simulink model "chap6_8sim"  (Simulink 5.0)
settings: Solver=ode45  StartTime=0.0  StopTime=20  RelTol=1e-3
libraries: simulink x1
settings Model: LastModifiedBy=Administrator

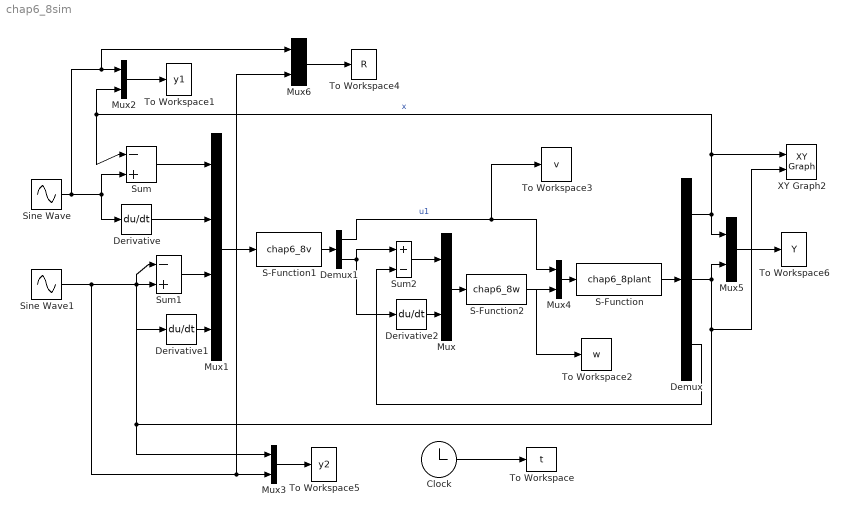
== system chap6_8sim ==
  Clock : Clock
  Demux : Demux  Outputs=3
  Demux1 : Demux  Outputs=2
  Derivative : Derivative
  Derivative1 : Derivative
  Derivative2 : Derivative
  Mux{,2..6} (6 alike) : Mux  Inputs=2
  Mux1 : Mux
  S-Function : S-Function  FunctionName=chap6_8plant  Parameters=state
  S-Function1 : S-Function  FunctionName=chap6_8v
  S-Function2 : S-Function  FunctionName=chap6_8w
  Sine Wave : Sin  Phase=pi/2  SampleTime=0
  Sine Wave1 : Sin  SampleTime=0
  Sum : Sum  Inputs=|-+  SaturateOnIntegerOverflow=on
  Sum1 : Sum  Inputs=|-+  SaturateOnIntegerOverflow=on
  Sum2 : Sum  Inputs=|+-  SaturateOnIntegerOverflow=on
  To Workspace : ToWorkspace  VariableName=t  SampleTime=-1  SaveFormat=Array
  To Workspace1 : ToWorkspace  VariableName=y1  SampleTime=-1  SaveFormat=Array
  To Workspace2 : ToWorkspace  VariableName=w  SampleTime=-1  SaveFormat=Array
  To Workspace3 : ToWorkspace  VariableName=v  SampleTime=-1  SaveFormat=Array
  To Workspace4 : ToWorkspace  VariableName=R  SampleTime=-1  SaveFormat=Array
  To Workspace5 : ToWorkspace  VariableName=y2  SampleTime=-1  SaveFormat=Array
  To Workspace6 : ToWorkspace  VariableName=Y  SampleTime=-1  SaveFormat=Array
  XY Graph2 : simulink/Sinks/XY Graph  xmin=-1.5  xmax=1.5  ymin=-1.5  ymax=1.5  st=-1
  wires:
  S-Function/1 -> Demux/1
  Demux/1 -> Mux5/1, Sum/1, Mux2/2, XY Graph2/1  "x"
  Mux1/1 -> S-Function1/1
  Demux/2 -> Mux5/2, Mux3/1, Sum1/1, XY Graph2/2
  Sine Wave/1 -> Derivative/1, Sum/2, Mux2/1, Mux6/1
  Sum1/1 -> Mux1/3
  Sine Wave1/1 -> Sum1/2, Derivative1/1, Mux3/2, Mux6/2
  Derivative/1 -> Mux1/2
  Derivative1/1 -> Mux1/4
  S-Function1/1 -> Demux1/1
  Sum/1 -> Mux1/1
  Demux1/2 -> Derivative2/1, Sum2/1
  Mux/1 -> S-Function2/1
  Mux2/1 -> To Workspace1/1
  Mux3/1 -> To Workspace5/1
  S-Function2/1 -> To Workspace2/1, Mux4/2
  Demux1/1 -> Mux4/1, To Workspace3/1  "u1"
  Mux4/1 -> S-Function/1
  Derivative2/1 -> Mux/2
  Clock/1 -> To Workspace/1
  Demux/3 -> Sum2/2
  Sum2/1 -> Mux/1
  Mux5/1 -> To Workspace6/1
  Mux6/1 -> To Workspace4/1
